simulink model "slexMulticoreFcn2"  (R2017b)
settings: Solver=FixedStepDiscrete  StartTime=0.0  StopTime=100  FixedStep=.2  RelTol=1e-3  EnableMultiTasking=on
Description:
  | Algorithm Design
settings Model: ParamWorkspaceSource=ReferencedWorkspace  ExtModeTrigMode=oneshot  ExtModeArmWhenConnect=off  ExtModeAutoUpdateStatusClock=off  Creator=The MathWorks, Inc.  LastModifiedBy=The MathWorks, Inc.
settings SolverCC: ConcurrentTasks=on
settings DataIOCC: SaveFormat=StructureWithTime  SaveOutput=off  SaveTime=off  SignalLoggingName=sigsOut
settings OptimizationCC: BlockReduction=off  DefaultParameterBehavior=Inlined  UseDivisionForNetSlopeComputation=UseDivisionForReciprocalsOfIntegersOnly  InlineInvariantSignals=on  EnhancedBackFolding=on  ExpressionDepthLimit=2147483647  StateBitsets=on  DataBitsets=on  EfficientFloat2IntCast=on  LifeSpan=inf  BufferReusableBoundary=off
settings DebuggingCC: UnderspecifiedInitializationDetection=Classic  MergeDetectMultiDrivingBlocksExec=none  CheckExecutionContextPreStartOutputMsg=on  CheckExecutionContextRuntimeOutputMsg=on  IntegerOverflowMsg=none  FcnCallInpInsideContextMsg=warning  AllowSymbolicDim=off  StateNameClashWarn=warning  StrictBusMsg=ErrorOnBusTreatedAsVector  SFUnexpectedBacktrackingDiag=warning  SFNoUnconditionalDefaultTransitionDiag=warning  SFExecutionAtInitializationDiag=none  IntegerSaturationMsg=none
settings HardwareCC: ProdBitPerLong=64  ProdBitPerPointer=32  ProdBitPerSizeT=32  ProdBitPerPtrDiffT=32  ProdLargestAtomicFloat=None  ProdLongLongMode=on  ProdHWDeviceType=Specified  TargetHWDeviceType=Generic->32-bit Embedded Processor
settings ModelReferenceCC: UpdateModelReferenceTargets=IfOutOfDate  ModelReferenceMinAlgLoopOccurrences=on  PropagateSignalLabelsOutOfModel=off
settings RTWCC: TLCOptions=-p0 -aWarnNonSaturatedBlocks=0  Description=Generic Real-Time Target  GenerateReport=on  RTWVerbose=off  LaunchReport=on
settings CodeAppCC: ForceParamTrailComments=on  MaxIdLength=64  StateflowObjectComments=on
settings GRTTargetCC: TargetLangStandard=C89/C90 (ANSI)  UtilityFuncGeneration=Shared location  GeneratePreprocessorConditionals=Disable all  CombineOutputUpdateFcns=off  MatFileLogging=off  SupportNonFinite=off
settings ConfigComp: CovMetricSettings=d  CovHtmlReporting=on  CovSaveCumulativeToWorkspaceVar=on  CovSaveSingleToWorkspaceVar=on  CovExternalEMLEnable=off  CovSFcnEnable=off

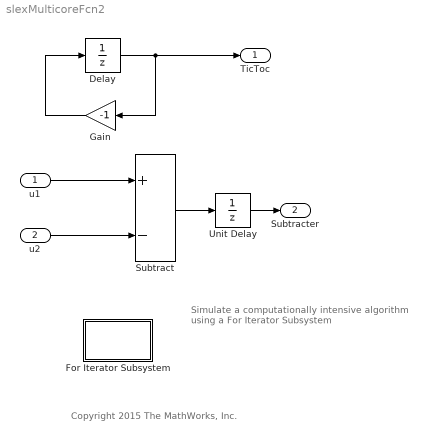
== system slexMulticoreFcn2 ==
  note: Simulate a computationally intensive algorithm using a For Iterator Subsystem
  note: Copyright 2015 The MathWorks, Inc.
  u1 : Inport  SampleTime=.2
  u2 : Inport  Port=2
  Delay : UnitDelay  InitialCondition=1  SampleTime=.4
  For Iterator Subsystem : Subsystem  TreatAsAtomicUnit=on
  Gain : Gain  Gain=-1  OutDataTypeStr=fixdt(1,8,0)
  Subtract : Sum  Inputs=+-
  Unit Delay : UnitDelay  SampleTime=-1
  TicToc : Outport  InitialOutput=0
  Subtracter : Outport  Port=2  InitialOutput=0
  wires:
  u2/1 -> Subtract/2
  u1/1 -> Subtract/1
  Delay/1 -> Gain/1, TicToc/1
  Gain/1 -> Delay/1
  Subtract/1 -> Unit Delay/1
  Unit Delay/1 -> Subtracter/1

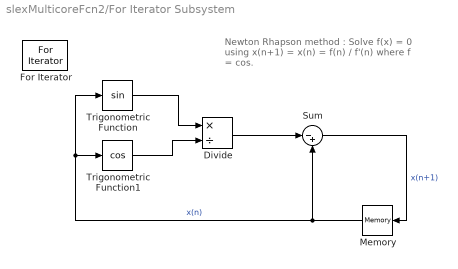
== system slexMulticoreFcn2/For Iterator Subsystem ==
  note: Newton Rhapson method :
      | Solve f(x) = 0 using
      | x(n+1) = x(n) = f(n) / f'(n) where f = cos.
  Divide : Product  Inputs=*/
  For Iterator : ForIterator  IterationLimit=nIter  ShowIterationPort=off
  Memory : Memory  InheritSampleTime=on
  Sum : Sum  Inputs=|-+
  Trigonometric Function : Trigonometry
  Trigonometric Function1 : Trigonometry  Operator=cos
  wires:
  Sum/1 -> Memory/1  "x(n+1)"
  Divide/1 -> Sum/1
  Trigonometric Function1/1 -> Divide/2
  Trigonometric Function/1 -> Divide/1
  Memory/1 -> Trigonometric Function/1, Trigonometric Function1/1, Sum/2  "x(n)"
